simulink model "harerev"  (Simulink 8.5)
settings: Solver=ode23s  SolverMode=SingleTasking  StartTime=0.0  StopTime=8.0  RelTol=1e-5  AbsTol=1e-8
values from neighbouring files (symbols this model uses):
  a1 = 5    [linmodharerev.m]
  a2 = 0.8    [linmodharerev.m]
  c1 = 0.05    [linmodharerev.m]
  c2 = 8e-5    (= 8e-05)    [linmodharerev.m]
  start_harer = l_hare*1.2    (= 12000)    [linmodharerev.m]
  start_rever = l_rev*0.2    (= 20)    [linmodharerev.m]
settings Model: Creator=bragerug  LastModifiedBy=ewilthil
settings DataIOCC: MaxDataPoints=10000
settings OptimizationCC: BlockReduction=off  BooleanDataType=off
settings DebuggingCC: SaveWithParameterizedLinksMsg=none  SignalResolutionControl=TryResolveAllWithWarning  MultiTaskDSMMsg=warning  MultiTaskCondExecSysMsg=none  FcnCallInpInsideContextMsg=UseLocalSettings
settings HardwareCC: TargetUnknown=on
settings RTWCC: TemplateMakefile=grt_vc.tmf

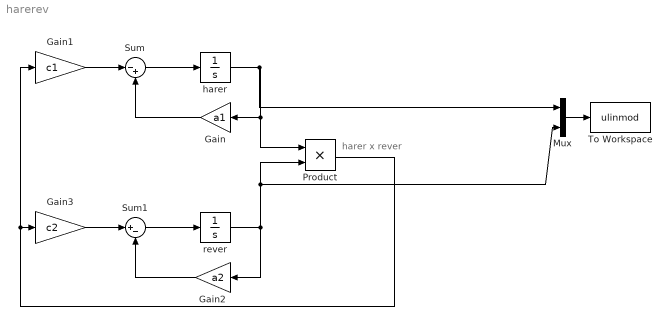
== system harerev ==
  note: harer x rever
  Gain : Gain  Gain=a1  SaturateOnIntegerOverflow=on  OutDataTypeStr=Inherit: Same as input  ParamDataTypeStr=Inherit: Same as input
  Gain1 : Gain  Gain=c1  SaturateOnIntegerOverflow=on  OutDataTypeStr=Inherit: Same as input  ParamDataTypeStr=Inherit: Same as input
  Gain2 : Gain  Gain=a2  SaturateOnIntegerOverflow=on  OutDataTypeStr=Inherit: Same as input  ParamDataTypeStr=Inherit: Same as input
  Gain3 : Gain  Gain=c2  SaturateOnIntegerOverflow=on  OutDataTypeStr=Inherit: Same as input  ParamDataTypeStr=Inherit: Same as input
  Mux : Mux  Inputs=2
  Product : Product  SaturateOnIntegerOverflow=on  RndMeth=Zero  InputSameDT=on  OutDataTypeStr=Inherit: Same as first input
  Sum : Sum  Inputs=|-+
  Sum1 : Sum  Inputs=|+-
  To Workspace : ToWorkspace  VariableName=ulinmod  SaveFormat=Timeseries  SampleTime=-1
  harer : Integrator  InitialCondition=start_harer
  rever : Integrator  InitialCondition=start_rever
  wires:
  rever/1 -> Mux/2, Product/2, Gain2/1
  harer/1 -> Mux/1, Product/1, Gain/1
  Gain2/1 -> Sum1/2
  Gain/1 -> Sum/2
  Sum/1 -> harer/1
  Sum1/1 -> rever/1
  Product/1 -> Gain1/1, Gain3/1
  Gain3/1 -> Sum1/1
  Gain1/1 -> Sum/1
  Mux/1 -> To Workspace/1
